simulink model "SingleInverterInfBus"  (R2020b)
settings: Solver=FixedStepAuto  StartTime=0.0  StopTime=20  FixedStep=Ts  RelTol=1e-3
values from neighbouring files (symbols this model uses):
  Cdc = 0.125    [Para.m]    (also in Para_VFM_FFL_Inverter.m = 0.101859163579; Para_VFM_FFL_Inverter_v2.m = 0.101859163579)
  Cf = 0.02    [Para.m]    (also in Para_VFM_FFL_Inverter.m; Para_VFM_FFL_Inverter_v2.m)
  Lc = 0.02    [Para.m]    (also in Para_VFM_FFL_Inverter.m; Para_VFM_FFL_Inverter_v2.m)
  Lf = 0.05    [Para.m]    (also in Para_VFM_FFL_Inverter.m; Para_VFM_FFL_Inverter_v2.m)
  m = 5/100    (= 0.05)    [Para.m]    (also in Para_VFM_FFL_Inverter.m; Para_VFM_FFL_Inverter_v2.m)
  Rline = Xline/5    (= 0.19)    [Para.m]    (also in Para_VFM_FFL_Inverter.m; Para_VFM_FFL_Inverter_v2.m)
  Sbase = 1    [Para.m]    (also in Para_VFM_FFL_Inverter.m; Para_VFM_FFL_Inverter_v2.m)
  Ts = 1/Fs    (= 0.0001)    [Para.m]    (also in Para_VFM_FFL_Inverter.m; Para_VFM_FFL_Inverter_v2.m = 5e-05)
  Vbase = 1    [Para.m]    (also in Para_VFM_FFL_Inverter.m; Para_VFM_FFL_Inverter_v2.m)
  vdc_ref = 2.5    [Para.m]    (also in Para_VFM_FFL_Inverter.m; Para_VFM_FFL_Inverter_v2.m)
  w_droop = 1*2*pi    (= 6.28318530718)    [Para.m]    (also in Para_VFM_FFL_Inverter.m = 31.4159265359; Para_VFM_FFL_Inverter_v2.m = 31.4159265359)
  w_i = 600*2*pi    (= 3769.91118431)    [Para.m]    (also in Para_VFM_FFL_Inverter.m; Para_VFM_FFL_Inverter_v2.m)
  w_pll = 15*2*pi    (= 94.2477796077)    [Para.m]    (also in Para_VFM_FFL_Inverter.m; Para_VFM_FFL_Inverter_v2.m)
  w_tau = 200*2*pi    (= 1256.63706144)    [Para.m]    (also in Para_VFM_FFL_Inverter.m; Para_VFM_FFL_Inverter_v2.m)
  w_v = 300*2*pi    (= 1884.95559215)    [Para.m]    (also in Para_VFM_FFL_Inverter.m; Para_VFM_FFL_Inverter_v2.m)
  w_vdc = 5*2*pi    (= 31.4159265359)    [Para.m]    (also in Para_VFM_FFL_Inverter.m; Para_VFM_FFL_Inverter_v2.m)
  Wbase = 2*pi*50    (= 314.159265359)    [Para.m]    (also in Para_VFM_FFL_Inverter.m; Para_VFM_FFL_Inverter_v2.m)
  Xline = 0.95    [Para.m]    (also in Para_VFM_FFL_Inverter.m; Para_VFM_FFL_Inverter_v2.m)
  Zbase = Vbase/Ibase    (= 1)    [Para.m]    (also in Para_VFM_FFL_Inverter.m; Para_VFM_FFL_Inverter_v2.m)
undefined symbols (not defined in the file or in its folder): DiscIntNeverNeededParam, initial
libraries: powerlib x282, SimplusGT x7
(part 3 of 8)

== system SingleInverterInfBus/Subsystem3 ==
  In1 : Inport
  Constant : Constant  Value=pi/2
  Constant2 : Constant  Value=2*pi
  Math Function1 : Math  Operator=mod  SignedPower=on  SaturateOnIntegerOverflow=on
  Sum1 : Sum  Inputs=|+-
  Sum3 : Sum  Inputs=|++
  Out1 : Outport
  wires:
  Sum3/1 -> Math Function1/1
  Constant2/1 -> Math Function1/2
  In1/1 -> Sum3/1
  Constant/1 -> Sum3/2, Sum1/2
  Math Function1/1 -> Sum1/1
  Sum1/1 -> Out1/1

== system SingleInverterInfBus/Subsystem4 ==
  In1 : Inport
  Constant : Constant  Value=pi/2
  Constant2 : Constant  Value=2*pi
  Math Function1 : Math  Operator=mod  SignedPower=on  SaturateOnIntegerOverflow=on
  Sum1 : Sum  Inputs=|+-
  Sum3 : Sum  Inputs=|++
  Out1 : Outport
  wires:
  Sum3/1 -> Math Function1/1
  Constant2/1 -> Math Function1/2
  In1/1 -> Sum3/1
  Constant/1 -> Sum1/2, Sum3/2
  Math Function1/1 -> Sum1/1
  Sum1/1 -> Out1/1

== system SingleInverterInfBus/Subsystem5 ==
  In1 : Inport
  Transfer Fcn : TransferFcn  Numerator=[1 0 0]  Denominator=[1 kp ki]
  Out1 : Outport
  wires:
  Transfer Fcn/1 -> Out1/1
  In1/1 -> Transfer Fcn/1

== system SingleInverterInfBus/Subsystem6 ==
  In1 : Inport
  Transfer Fcn : TransferFcn  Numerator=[1 kd*ki 0]  Denominator=[1 kd*ki ki]
  Out1 : Outport
  wires:
  Transfer Fcn/1 -> Out1/1
  In1/1 -> Transfer Fcn/1

== system SingleInverterInfBus/Subsystem7 ==
  In1 : Inport
  Transfer Fcn : TransferFcn  Numerator=[1 0]  Denominator=[1 kp ki]
  Out1 : Outport
  wires:
  Transfer Fcn/1 -> Out1/1
  In1/1 -> Transfer Fcn/1

== system SingleInverterInfBus/Subsystem8 ==
  In1 : Inport
  Transfer Fcn : TransferFcn  Numerator=[1 kd*ki]  Denominator=[1 kd*ki ki]
  Out1 : Outport
  wires:
  Transfer Fcn/1 -> Out1/1
  In1/1 -> Transfer Fcn/1

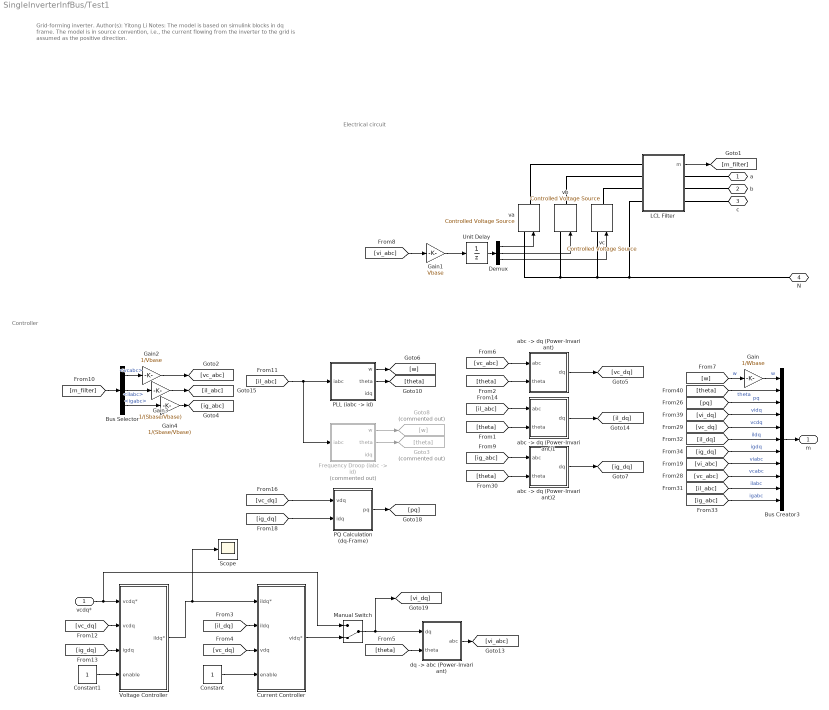
== system SingleInverterInfBus/Test1 ==
  note: Grid-forming inverter.
      |
      | Author(s): Yitong Li
      |
      | Notes:
      |
      | The model is based on simulink blocks in dq frame.
      |
      | The model is in source convention, i.e., the current flowing from the inverter to the grid is assumed as the positive direction.
  note: Electrical circuit
  note: Controller
  vcdq* : Inport
  Bus Creator3 : BusCreator  Inputs=11
  Bus Selector : BusSelector  OutputSignals=vcabc,ilabc,igabc
  Constant : Constant
  Constant1 : Constant
  Current Controller : Subsystem  mask{Ts=Ts, Wbase=Wbase, Lf=Lf/Wbase, Kg=0, Kp=w_i*Lf/Wbase, Ki=w_i*w_i/4*Lf/Wbase, xdmax=inf, xqmax=inf, Kcd=0}
      mask prompts: Ts "Sampling Time (s)"; Wbase "Base Angular Frequency (rad/s)"; Lf "Inductance"; Kg "Estimator Gain"; Kp "Proportional Gain"; Ki "Integral Gain"; xdmax "Voltage D Limit"; xqmax "Voltage Q Limit"; Kcd "Cross Decoupling Gain"
  Demux : Demux  Outputs=3
  "Frequency Droop (iabc -> id)" : Subsystem  Commented=on  AncestorBlock=|  mask{Ts=Ts, Sbase=Sbase, Vbase=Vbase, Wbase=Wbase, m=5/100, w_tau=15*2*pi, theta0=0, i0=0, w0=1}
      | SimplusGT/Frequency Droop
      | (iabc -> id)
      mask prompts: Ts "Ts (s), samping period"; Sbase "Sbase (VA), base power"; Vbase "Vbase (V), base voltage"; Wbase "Wbase (rad/s), base angular frequency"; m "m (pu), droop gain"; w_tau "w_tau (rad/s), low-pass filter bandwidth"; theta0 "theta0 (rad), initial angle"; i0 "i0 (pu), current setting point"; w0 "w0 (pu), frequency setting point"
  Gain : Gain  Gain=1/Wbase
  Gain1 : Gain  Gain=Vbase
  Gain2 : Gain  Gain=1/Vbase
  Gain3 : Gain  Gain=1/(Sbase/Vbase)
  Gain4 : Gain  Gain=1/(Sbase/Vbase)
  Goto3 : Goto  Commented=on  GotoTag=theta
  Goto8 : Goto  Commented=on  GotoTag=w
  LCL Filter : Subsystem  AncestorBlock=SimplexPS/LCL Filter  mask{Lf=Lf*(Vbase^2/Sbase)/Wbase, Rf=Lf*(Vbase^2/Sbase)/5, Lc=Lc*(Vbase^2/Sbase)/Wbase, Rc=Lc*(Vbase^2/Sbase)/5, Cf=Cf*(Sbase/Vbase^2)/Wbase, Rd=1e-5*(Vbase^2/Sbase)}
      mask prompts: Lf "Lf (H)"; Rf "Rf (Ohm)"; Lc "Lc (H)"; Rc "Rc (Ohm)"; Cf "Cf (F)"; Rd "Rd (Ohm)"
  Manual Switch : ManualSwitch  CurrentSetting=0
  "PLL (iabc -> id)" : Subsystem  mask{Ts=Ts, Ibase=Sbase/Vbase, Wbase=Wbase, w_pll=0, w_tau=0, theta0=0}
      mask prompts: Ts "Ts (s), sampling period"; Ibase "Ibase (V), base current"; Wbase "Wbase (rad/s), base angular frequency"; w_pll "w_pll (rad/s), PLL bandwidth"; w_tau "w_tau (rad/s), low-pass filter bandwidth"; theta0 "theta0 (rad), initial angle"
  PQ Calculation (dq-Frame) : Subsystem  AncestorBlock=|
      | SimplusGT/PQ Calculation
      | (dq-Frame)
  Scope : Scope
  Unit Delay : UnitDelay  SampleTime=-1  HasFrameUpgradeWarning=on
  Voltage Controller : Subsystem  mask{Ts=Ts, Wbase=Wbase, Cf=Cf/Wbase, Kg=0, Kp=w_v*Cf/Wbase, Ki=w_v*w_v/4*Cf/Wbase*50, xdmax=inf, xqmax=inf, Kcd=0}
      mask prompts: Ts "Sampling Time (s)"; Wbase "Base Angular Frequency (rad/s)"; Cf "Capacitance"; Kg "Estimator Gain"; Kp "Proportional Gain"; Ki "Integral Gain"; xdmax "Current D Limit"; xqmax "Current Q Limit"; Kcd "Cross Decoupling Gain"
  "abc -> dq (Power-Invariant)" : Subsystem  AncestorBlock=|
      | SimplusGT/abc -> dq
      | (Power-Invariant)
  "abc -> dq (Power-Invariant)1" : Subsystem  AncestorBlock=|
      | SimplusGT/abc -> dq
      | (Power-Invariant)
  "abc -> dq (Power-Invariant)2" : Subsystem  AncestorBlock=|
      | SimplusGT/abc -> dq
      | (Power-Invariant)
  "dq -> abc (Power-Invariant)" : Subsystem  AncestorBlock=|
      | SimplusGT/dq -> abc
      | (Power-Invariant)
  va : powerlib/Electrical Sources/Controlled Voltage Source  Initialize=on  Source_Type=AC  Amplitude=0  Phase=0  Frequency=0  Measurements=None
  vb : powerlib/Electrical Sources/Controlled Voltage Source  Initialize=on  Source_Type=AC  Amplitude=0  Phase=0  Frequency=0  Measurements=None
  vc : powerlib/Electrical Sources/Controlled Voltage Source  Initialize=on  Source_Type=AC  Amplitude=0  Phase=0  Frequency=0  Measurements=None
  a : PMIOPort  Side=Right
  b : PMIOPort  Port=2  Side=Right
  c : PMIOPort  Port=3  Side=Right
  N : PMIOPort  Port=4  Side=Right
  m : Outport
  wires:
  Gain1/1 -> Unit Delay/1
  [vi_abc] -> Gain1/1
  Gain4/1 -> [ig_abc]
  Gain3/1 -> [il_abc]
  Gain2/1 -> [vc_abc]
  [ig_dq] -> Voltage Controller/3(igdq)
  [vc_dq] -> Voltage Controller/2(vcdq)
  Constant1/1 -> Voltage Controller/4(enable)
  Voltage Controller/1(ildq*) -> Scope/1, Current Controller/1(iIdq*)
  vcdq*/1 -> Manual Switch/1, Voltage Controller/1(vcdq*)
  [ig_abc] -> Bus Creator3/11  "igabc"
  [il_abc] -> Bus Creator3/10  "ilabc"
  [vc_abc] -> Bus Creator3/9  "vcabc"
  [vi_abc] -> Bus Creator3/8  "viabc"
  [ig_dq] -> Bus Creator3/7  "igdq"
  [il_dq] -> Bus Creator3/6  "ildq"
  [vc_dq] -> Bus Creator3/5  "vcdq"
  [vi_dq] -> Bus Creator3/4  "vidq"
  [pq] -> Bus Creator3/3  "pq"
  [theta] -> Bus Creator3/2  "theta"
  Gain/1 -> Bus Creator3/1  "w"
  [w] -> Gain/1  "w"
  Bus Selector/1 -> Gain2/1  "<vcabc>"
  Unit Delay/1 -> Demux/1
  [m_filter] -> Bus Selector/1
  "abc -> dq (Power-Invariant)1"/1(dq) -> [il_dq]
  "abc -> dq (Power-Invariant)2"/1(dq) -> [ig_dq]
  "abc -> dq (Power-Invariant)"/1(dq) -> [vc_dq]
  [il_dq] -> Current Controller/2(iIdq)
  [ig_dq] -> PQ Calculation (dq-Frame)/2(idq)
  PQ Calculation (dq-Frame)/1(pq) -> [pq]
  [vc_dq] -> PQ Calculation (dq-Frame)/1(vdq)
  [theta] -> "dq -> abc (Power-Invariant)"/2(theta)
  [vc_dq] -> Current Controller/3(vdq)
  Constant/1 -> Current Controller/4(enable)
  Bus Selector/2 -> Gain3/1  "<ilabc>"
  Bus Selector/3 -> Gain4/1  "<igabc>"
  [theta] -> "abc -> dq (Power-Invariant)2"/2(theta)
  [ig_abc] -> "abc -> dq (Power-Invariant)2"/1(abc)
  [il_abc] -> "abc -> dq (Power-Invariant)1"/1(abc)
  [vc_abc] -> "abc -> dq (Power-Invariant)"/1(abc)
  [theta] -> "abc -> dq (Power-Invariant)1"/2(theta)
  [theta] -> "abc -> dq (Power-Invariant)"/2(theta)
  Demux/3 -> vc/1
  Demux/2 -> vb/1
  Demux/1 -> va/1
  LCL Filter/1(m) -> [m_filter]
  Bus Creator3/1 -> m/1
  "dq -> abc (Power-Invariant)"/1(abc) -> [vi_abc]
  Current Controller/1(vidq*) -> Manual Switch/2
  Manual Switch/1 -> [vi_dq], "dq -> abc (Power-Invariant)"/1(dq)
  "PLL (iabc -> id)"/1(w) -> [w]
  "PLL (iabc -> id)"/2(theta) -> [theta]
  [il_abc] -> "Frequency Droop (iabc -> id)"/1(iabc), "PLL (iabc -> id)"/1(iabc)
  "Frequency Droop (iabc -> id)"/1(w) -> Goto8/1
  "Frequency Droop (iabc -> id)"/2(theta) -> Goto3/1
  connections:
  LCL Filter/LConn3 -- vc/RConn1
  va/LConn1 -- vb/LConn1 -- vc/LConn1 -- LCL Filter/LConn4 -- N/RConn1
  LCL Filter/RConn3 -- c/RConn1
  LCL Filter/RConn2 -- b/RConn1
  LCL Filter/RConn1 -- a/RConn1
  LCL Filter/LConn1 -- va/RConn1
  LCL Filter/LConn2 -- vb/RConn1

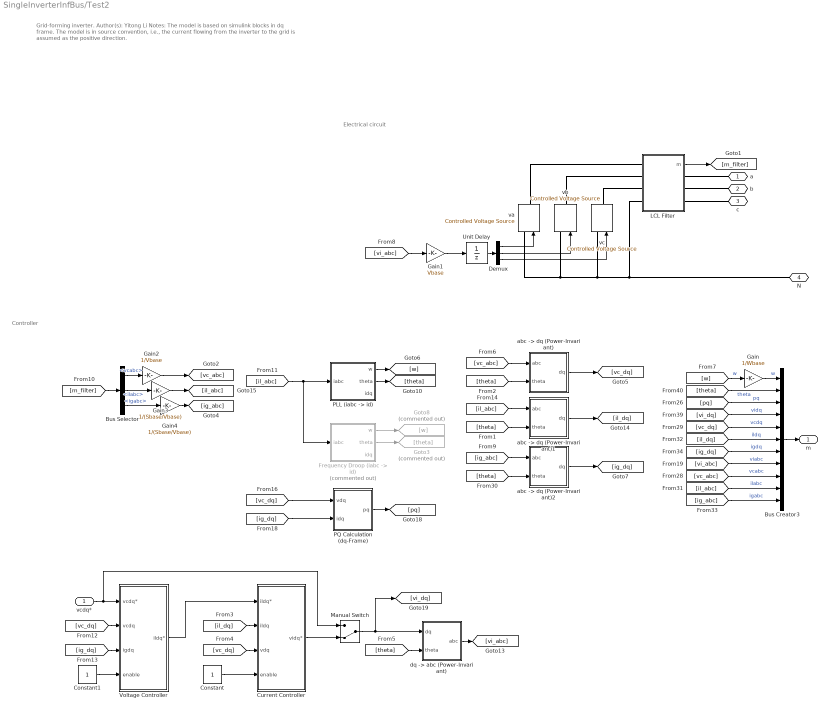
== system SingleInverterInfBus/Test2 ==
  note: Grid-forming inverter.
      |
      | Author(s): Yitong Li
      |
      | Notes:
      |
      | The model is based on simulink blocks in dq frame.
      |
      | The model is in source convention, i.e., the current flowing from the inverter to the grid is assumed as the positive direction.
  note: Electrical circuit
  note: Controller
  vcdq* : Inport
  Bus Creator3 : BusCreator  Inputs=11
  Bus Selector : BusSelector  OutputSignals=vcabc,ilabc,igabc
  Constant : Constant
  Constant1 : Constant
  Current Controller : Subsystem  mask{Ts=Ts, Wbase=Wbase, Lf=Lf/Wbase, Kg=0, Kp=w_i*Lf/Wbase, Ki=w_i*w_i/4*Lf/Wbase, xdmax=inf, xqmax=inf, Kcd=0}
      mask prompts: Ts "Sampling Time (s)"; Wbase "Base Angular Frequency (rad/s)"; Lf "Inductance"; Kg "Estimator Gain"; Kp "Proportional Gain"; Ki "Integral Gain"; xdmax "Voltage D Limit"; xqmax "Voltage Q Limit"; Kcd "Cross Decoupling Gain"
  Demux : Demux  Outputs=3
  "Frequency Droop (iabc -> id)" : Subsystem  Commented=on  AncestorBlock=|  mask{Ts=Ts, Sbase=Sbase, Vbase=Vbase, Wbase=Wbase, m=5/100, w_tau=15*2*pi, theta0=0, i0=0, w0=1}
      | SimplusGT/Frequency Droop
      | (iabc -> id)
      mask prompts: Ts "Ts (s), samping period"; Sbase "Sbase (VA), base power"; Vbase "Vbase (V), base voltage"; Wbase "Wbase (rad/s), base angular frequency"; m "m (pu), droop gain"; w_tau "w_tau (rad/s), low-pass filter bandwidth"; theta0 "theta0 (rad), initial angle"; i0 "i0 (pu), current setting point"; w0 "w0 (pu), frequency setting point"
  Gain : Gain  Gain=1/Wbase
  Gain1 : Gain  Gain=Vbase
  Gain2 : Gain  Gain=1/Vbase
  Gain3 : Gain  Gain=1/(Sbase/Vbase)
  Gain4 : Gain  Gain=1/(Sbase/Vbase)
  Goto3 : Goto  Commented=on  GotoTag=theta
  Goto8 : Goto  Commented=on  GotoTag=w
  LCL Filter : Subsystem  AncestorBlock=SimplexPS/LCL Filter  mask{Lf=Lf*(Vbase^2/Sbase)/Wbase, Rf=Lf*(Vbase^2/Sbase)/5, Lc=Lc*(Vbase^2/Sbase)/Wbase, Rc=Lc*(Vbase^2/Sbase)/5, Cf=Cf*(Sbase/Vbase^2)/Wbase, Rd=1e-5*(Vbase^2/Sbase)}
      mask prompts: Lf "Lf (H)"; Rf "Rf (Ohm)"; Lc "Lc (H)"; Rc "Rc (Ohm)"; Cf "Cf (F)"; Rd "Rd (Ohm)"
  Manual Switch : ManualSwitch  CurrentSetting=0
  "PLL (iabc -> id)" : Subsystem  mask{Ts=Ts, Ibase=Sbase/Vbase, Wbase=Wbase, w_pll=5*2*pi, w_tau=15*2*pi, theta0=0}
      mask prompts: Ts "Ts (s), sampling period"; Ibase "Ibase (V), base current"; Wbase "Wbase (rad/s), base angular frequency"; w_pll "w_pll (rad/s), PLL bandwidth"; w_tau "w_tau (rad/s), low-pass filter bandwidth"; theta0 "theta0 (rad), initial angle"
  PQ Calculation (dq-Frame) : Subsystem  AncestorBlock=|
      | SimplusGT/PQ Calculation
      | (dq-Frame)
  Unit Delay : UnitDelay  SampleTime=-1  HasFrameUpgradeWarning=on
  Voltage Controller : Subsystem  mask{Ts=Ts, Wbase=Wbase, Cf=Cf/Wbase, Kg=0, Kp=w_v*Cf/Wbase, Ki=w_v*w_v/4*Cf/Wbase*20, xdmax=inf, xqmax=inf, Kcd=0}
      mask prompts: Ts "Sampling Time (s)"; Wbase "Base Angular Frequency (rad/s)"; Cf "Capacitance"; Kg "Estimator Gain"; Kp "Proportional Gain"; Ki "Integral Gain"; xdmax "Current D Limit"; xqmax "Current Q Limit"; Kcd "Cross Decoupling Gain"
  "abc -> dq (Power-Invariant)" : Subsystem  AncestorBlock=|
      | SimplusGT/abc -> dq
      | (Power-Invariant)
  "abc -> dq (Power-Invariant)1" : Subsystem  AncestorBlock=|
      | SimplusGT/abc -> dq
      | (Power-Invariant)
  "abc -> dq (Power-Invariant)2" : Subsystem  AncestorBlock=|
      | SimplusGT/abc -> dq
      | (Power-Invariant)
  "dq -> abc (Power-Invariant)" : Subsystem  AncestorBlock=|
      | SimplusGT/dq -> abc
      | (Power-Invariant)
  va : powerlib/Electrical Sources/Controlled Voltage Source  Initialize=on  Source_Type=AC  Amplitude=0  Phase=0  Frequency=0  Measurements=None
  vb : powerlib/Electrical Sources/Controlled Voltage Source  Initialize=on  Source_Type=AC  Amplitude=0  Phase=0  Frequency=0  Measurements=None
  vc : powerlib/Electrical Sources/Controlled Voltage Source  Initialize=on  Source_Type=AC  Amplitude=0  Phase=0  Frequency=0  Measurements=None
  a : PMIOPort  Side=Right
  b : PMIOPort  Port=2  Side=Right
  c : PMIOPort  Port=3  Side=Right
  N : PMIOPort  Port=4  Side=Right
  m : Outport
  wires:
  Gain1/1 -> Unit Delay/1
  [vi_abc] -> Gain1/1
  Gain4/1 -> [ig_abc]
  Gain3/1 -> [il_abc]
  Gain2/1 -> [vc_abc]
  [ig_dq] -> Voltage Controller/3(igdq)
  [vc_dq] -> Voltage Controller/2(vcdq)
  Constant1/1 -> Voltage Controller/4(enable)
  Voltage Controller/1(ildq*) -> Current Controller/1(iIdq*)
  vcdq*/1 -> Manual Switch/1, Voltage Controller/1(vcdq*)
  [ig_abc] -> Bus Creator3/11  "igabc"
  [il_abc] -> Bus Creator3/10  "ilabc"
  [vc_abc] -> Bus Creator3/9  "vcabc"
  [vi_abc] -> Bus Creator3/8  "viabc"
  [ig_dq] -> Bus Creator3/7  "igdq"
  [il_dq] -> Bus Creator3/6  "ildq"
  [vc_dq] -> Bus Creator3/5  "vcdq"
  [vi_dq] -> Bus Creator3/4  "vidq"
  [pq] -> Bus Creator3/3  "pq"
  [theta] -> Bus Creator3/2  "theta"
  Gain/1 -> Bus Creator3/1  "w"
  [w] -> Gain/1  "w"
  Bus Selector/1 -> Gain2/1  "<vcabc>"
  Unit Delay/1 -> Demux/1
  [m_filter] -> Bus Selector/1
  "abc -> dq (Power-Invariant)1"/1(dq) -> [il_dq]
  "abc -> dq (Power-Invariant)2"/1(dq) -> [ig_dq]
  "abc -> dq (Power-Invariant)"/1(dq) -> [vc_dq]
  [il_dq] -> Current Controller/2(iIdq)
  [ig_dq] -> PQ Calculation (dq-Frame)/2(idq)
  PQ Calculation (dq-Frame)/1(pq) -> [pq]
  [vc_dq] -> PQ Calculation (dq-Frame)/1(vdq)
  [theta] -> "dq -> abc (Power-Invariant)"/2(theta)
  [vc_dq] -> Current Controller/3(vdq)
  Constant/1 -> Current Controller/4(enable)
  Bus Selector/2 -> Gain3/1  "<ilabc>"
  Bus Selector/3 -> Gain4/1  "<igabc>"
  [theta] -> "abc -> dq (Power-Invariant)2"/2(theta)
  [ig_abc] -> "abc -> dq (Power-Invariant)2"/1(abc)
  [il_abc] -> "abc -> dq (Power-Invariant)1"/1(abc)
  [vc_abc] -> "abc -> dq (Power-Invariant)"/1(abc)
  [theta] -> "abc -> dq (Power-Invariant)1"/2(theta)
  [theta] -> "abc -> dq (Power-Invariant)"/2(theta)
  Demux/3 -> vc/1
  Demux/2 -> vb/1
  Demux/1 -> va/1
  LCL Filter/1(m) -> [m_filter]
  Bus Creator3/1 -> m/1
  "dq -> abc (Power-Invariant)"/1(abc) -> [vi_abc]
  Current Controller/1(vidq*) -> Manual Switch/2
  Manual Switch/1 -> [vi_dq], "dq -> abc (Power-Invariant)"/1(dq)
  "PLL (iabc -> id)"/1(w) -> [w]
  "PLL (iabc -> id)"/2(theta) -> [theta]
  [il_abc] -> "Frequency Droop (iabc -> id)"/1(iabc), "PLL (iabc -> id)"/1(iabc)
  "Frequency Droop (iabc -> id)"/1(w) -> Goto8/1
  "Frequency Droop (iabc -> id)"/2(theta) -> Goto3/1
  connections:
  LCL Filter/LConn3 -- vc/RConn1
  va/LConn1 -- vb/LConn1 -- vc/LConn1 -- LCL Filter/LConn4 -- N/RConn1
  LCL Filter/RConn3 -- c/RConn1
  LCL Filter/RConn2 -- b/RConn1
  LCL Filter/RConn1 -- a/RConn1
  LCL Filter/LConn1 -- va/RConn1
  LCL Filter/LConn2 -- vb/RConn1

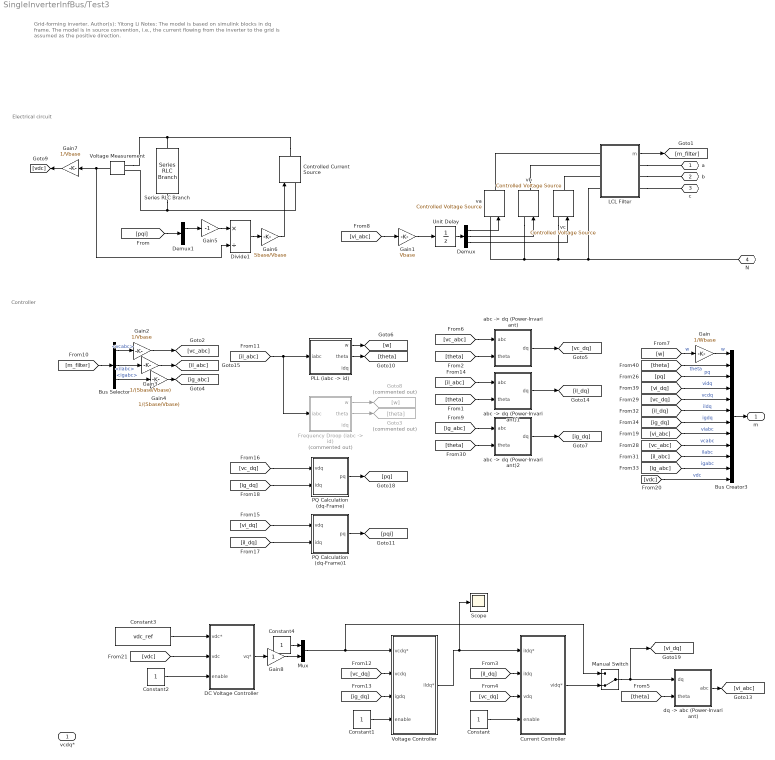
== system SingleInverterInfBus/Test3 ==
  note: Grid-forming inverter.
      |
      | Author(s): Yitong Li
      |
      | Notes:
      |
      | The model is based on simulink blocks in dq frame.
      |
      | The model is in source convention, i.e., the current flowing from the inverter to the grid is assumed as the positive direction.
  note: Electrical circuit
  note: Controller
  vcdq* : Inport
  Bus Creator3 : BusCreator  Inputs=12
  Bus Selector : BusSelector  OutputSignals=vcabc,ilabc,igabc
  Constant{,1..2,4} (4 alike) : Constant
  Constant3 : Constant  Value=vdc_ref
  Controlled Current Source : powerlib/Electrical Sources/Controlled Current Source  Initialize=on  Source_Type=AC  Amplitude=0  Phase=0  Frequency=0  Measurements=None
  Current Controller : Subsystem  mask{Ts=Ts, Wbase=Wbase, Lf=Lf/Wbase, Kg=0, Kp=w_i*Lf/Wbase, Ki=w_i*w_i/4*Lf/Wbase, xdmax=inf, xqmax=inf, Kcd=0}
      mask prompts: Ts "Sampling Time (s)"; Wbase "Base Angular Frequency (rad/s)"; Lf "Inductance"; Kg "Estimator Gain"; Kp "Proportional Gain"; Ki "Integral Gain"; xdmax "Voltage D Limit"; xqmax "Voltage Q Limit"; Kcd "Cross Decoupling Gain"
  DC Voltage Controller : Subsystem  mask{Ts=Ts, Wbase=Wbase, Kg=0, Kp=vdc_ref*Cdc*w_vdc, Ki=vdc_ref*Cdc*w_vdc^2/4}
      mask prompts: Ts "Sampling Time (s)"; Wbase "Base Angular Frequency (rad/s)"; Kg "Estimator Gain"; Kp "Proportional Gain"; Ki "Integral Gain"
  Demux : Demux  Outputs=3
  Demux1 : Demux  Outputs=2
  Divide1 : Product  Inputs=*/
  "Frequency Droop (iabc -> id)" : Subsystem  Commented=on  AncestorBlock=|  mask{Ts=Ts, Sbase=Sbase, Vbase=Vbase, Wbase=Wbase, m=5/100, w_tau=15*2*pi, theta0=0, i0=0, w0=1}
      | SimplusGT/Frequency Droop
      | (iabc -> id)
      mask prompts: Ts "Ts (s), samping period"; Sbase "Sbase (VA), base power"; Vbase "Vbase (V), base voltage"; Wbase "Wbase (rad/s), base angular frequency"; m "m (pu), droop gain"; w_tau "w_tau (rad/s), low-pass filter bandwidth"; theta0 "theta0 (rad), initial angle"; i0 "i0 (pu), current setting point"; w0 "w0 (pu), frequency setting point"
  Gain : Gain  Gain=1/Wbase
  Gain1 : Gain  Gain=Vbase
  Gain2 : Gain  Gain=1/Vbase
  Gain3 : Gain  Gain=1/(Sbase/Vbase)
  Gain4 : Gain  Gain=1/(Sbase/Vbase)
  Gain5 : Gain  Gain=-1
  Gain6 : Gain  Gain=Sbase/Vbase
  Gain7 : Gain  Gain=1/Vbase
  Gain8 : Gain
  Goto3 : Goto  Commented=on  GotoTag=theta
  Goto8 : Goto  Commented=on  GotoTag=w
  LCL Filter : Subsystem  AncestorBlock=SimplexPS/LCL Filter  mask{Lf=Lf*(Vbase^2/Sbase)/Wbase, Rf=Lf*(Vbase^2/Sbase)/5, Lc=Lc*(Vbase^2/Sbase)/Wbase, Rc=Lc*(Vbase^2/Sbase)/5, Cf=Cf*(Sbase/Vbase^2)/Wbase, Rd=1e-5*(Vbase^2/Sbase)}
      mask prompts: Lf "Lf (H)"; Rf "Rf (Ohm)"; Lc "Lc (H)"; Rc "Rc (Ohm)"; Cf "Cf (F)"; Rd "Rd (Ohm)"
  Manual Switch : ManualSwitch  CurrentSetting=0
  Mux : Mux  Inputs=2
  "PLL (iabc -> id)" : Subsystem  mask{Ts=Ts, Ibase=Sbase/Vbase, Wbase=Wbase, w_pll=0, w_tau=0, theta0=0}
      mask prompts: Ts "Ts (s), sampling period"; Ibase "Ibase (V), base current"; Wbase "Wbase (rad/s), base angular frequency"; w_pll "w_pll (rad/s), PLL bandwidth"; w_tau "w_tau (rad/s), low-pass filter bandwidth"; theta0 "theta0 (rad), initial angle"
  PQ Calculation (dq-Frame) : Subsystem  AncestorBlock=|
      | SimplusGT/PQ Calculation
      | (dq-Frame)
  PQ Calculation (dq-Frame)1 : Subsystem  AncestorBlock=|
      | SimplusGT/PQ Calculation
      | (dq-Frame)
  Scope : Scope
  Series RLC Branch : powerlib/Elements/Series RLC Branch  LConnTagsString=__new0  RConnTagsString=__new0  BranchType=RC  Resistance=1e-9*(Vbase^2/Sbase)  Inductance=1e-3  SetiL0=off  InitialCurrent=0  Capacitance=Cdc*(Sbase/Vbase^2)  Setx0=on  InitialVoltage=Vbase*vdc_ref  Measurements=None
  Unit Delay : UnitDelay  SampleTime=-1  HasFrameUpgradeWarning=on
  Voltage Controller : Subsystem  mask{Ts=Ts, Wbase=Wbase, Cf=Cf/Wbase, Kg=0, Kp=w_v*Cf/Wbase, Ki=w_v*w_v/4*Cf/Wbase*50, xdmax=inf, xqmax=inf, Kcd=0}
      mask prompts: Ts "Sampling Time (s)"; Wbase "Base Angular Frequency (rad/s)"; Cf "Capacitance"; Kg "Estimator Gain"; Kp "Proportional Gain"; Ki "Integral Gain"; xdmax "Current D Limit"; xqmax "Current Q Limit"; Kcd "Cross Decoupling Gain"
  Voltage Measurement : powerlib/Measurements/Voltage Measurement  PhasorSimulation=off  OutputType=Complex  PSBequivalent=0
  "abc -> dq (Power-Invariant)" : Subsystem  AncestorBlock=|
      | SimplusGT/abc -> dq
      | (Power-Invariant)
  "abc -> dq (Power-Invariant)1" : Subsystem  AncestorBlock=|
      | SimplusGT/abc -> dq
      | (Power-Invariant)
  "abc -> dq (Power-Invariant)2" : Subsystem  AncestorBlock=|
      | SimplusGT/abc -> dq
      | (Power-Invariant)
  "dq -> abc (Power-Invariant)" : Subsystem  AncestorBlock=|
      | SimplusGT/dq -> abc
      | (Power-Invariant)
  va : powerlib/Electrical Sources/Controlled Voltage Source  Initialize=on  Source_Type=AC  Amplitude=0  Phase=0  Frequency=0  Measurements=None
  vb : powerlib/Electrical Sources/Controlled Voltage Source  Initialize=on  Source_Type=AC  Amplitude=0  Phase=0  Frequency=0  Measurements=None
  vc : powerlib/Electrical Sources/Controlled Voltage Source  Initialize=on  Source_Type=AC  Amplitude=0  Phase=0  Frequency=0  Measurements=None
  a : PMIOPort  Side=Right
  b : PMIOPort  Port=2  Side=Right
  c : PMIOPort  Port=3  Side=Right
  N : PMIOPort  Port=4  Side=Right
  m : Outport
  wires:
  Gain1/1 -> Unit Delay/1
  [vi_abc] -> Gain1/1
  Gain4/1 -> [ig_abc]
  Gain3/1 -> [il_abc]
  Gain2/1 -> [vc_abc]
  [ig_dq] -> Voltage Controller/3(igdq)
  [vc_dq] -> Voltage Controller/2(vcdq)
  Constant1/1 -> Voltage Controller/4(enable)
  Voltage Controller/1(ildq*) -> Scope/1, Current Controller/1(iIdq*)
  [ig_abc] -> Bus Creator3/11  "igabc"
  [il_abc] -> Bus Creator3/10  "ilabc"
  [vc_abc] -> Bus Creator3/9  "vcabc"
  [vi_abc] -> Bus Creator3/8  "viabc"
  [ig_dq] -> Bus Creator3/7  "igdq"
  [il_dq] -> Bus Creator3/6  "ildq"
  [vc_dq] -> Bus Creator3/5  "vcdq"
  [vi_dq] -> Bus Creator3/4  "vidq"
  [pq] -> Bus Creator3/3  "pq"
  [theta] -> Bus Creator3/2  "theta"
  Gain/1 -> Bus Creator3/1  "w"
  [w] -> Gain/1  "w"
  Bus Selector/1 -> Gain2/1  "<vcabc>"
  Unit Delay/1 -> Demux/1
  [m_filter] -> Bus Selector/1
  "abc -> dq (Power-Invariant)1"/1(dq) -> [il_dq]
  "abc -> dq (Power-Invariant)2"/1(dq) -> [ig_dq]
  "abc -> dq (Power-Invariant)"/1(dq) -> [vc_dq]
  [il_dq] -> Current Controller/2(iIdq)
  [ig_dq] -> PQ Calculation (dq-Frame)/2(idq)
  PQ Calculation (dq-Frame)/1(pq) -> [pq]
  [vc_dq] -> PQ Calculation (dq-Frame)/1(vdq)
  [theta] -> "dq -> abc (Power-Invariant)"/2(theta)
  [vc_dq] -> Current Controller/3(vdq)
  Constant/1 -> Current Controller/4(enable)
  Bus Selector/2 -> Gain3/1  "<ilabc>"
  Bus Selector/3 -> Gain4/1  "<igabc>"
  [theta] -> "abc -> dq (Power-Invariant)2"/2(theta)
  [ig_abc] -> "abc -> dq (Power-Invariant)2"/1(abc)
  [il_abc] -> "abc -> dq (Power-Invariant)1"/1(abc)
  [vc_abc] -> "abc -> dq (Power-Invariant)"/1(abc)
  [theta] -> "abc -> dq (Power-Invariant)1"/2(theta)
  [theta] -> "abc -> dq (Power-Invariant)"/2(theta)
  Demux/3 -> vc/1
  Demux/2 -> vb/1
  Demux/1 -> va/1
  LCL Filter/1(m) -> [m_filter]
  Bus Creator3/1 -> m/1
  "dq -> abc (Power-Invariant)"/1(abc) -> [vi_abc]
  Current Controller/1(vidq*) -> Manual Switch/2
  Manual Switch/1 -> [vi_dq], "dq -> abc (Power-Invariant)"/1(dq)
  "PLL (iabc -> id)"/1(w) -> [w]
  "PLL (iabc -> id)"/2(theta) -> [theta]
  [il_abc] -> "Frequency Droop (iabc -> id)"/1(iabc), "PLL (iabc -> id)"/1(iabc)
  "Frequency Droop (iabc -> id)"/1(w) -> Goto8/1
  "Frequency Droop (iabc -> id)"/2(theta) -> Goto3/1
  Divide1/1 -> Gain6/1
  Gain6/1 -> Controlled Current Source/1
  Gain7/1 -> [vdc]
  Demux1/1 -> Gain5/1
  Gain5/1 -> Divide1/1
  [pqi] -> Demux1/1
  Voltage Measurement/1 -> Gain7/1, Divide1/2
  PQ Calculation (dq-Frame)1/1(pq) -> [pqi]
  [il_dq] -> PQ Calculation (dq-Frame)1/2(idq)
  [vi_dq] -> PQ Calculation (dq-Frame)1/1(vdq)
  Constant4/1 -> Mux/1
  DC Voltage Controller/1(vq*) -> Gain8/1
  Gain8/1 -> Mux/2
  Constant2/1 -> DC Voltage Controller/3(enable)
  Constant3/1 -> DC Voltage Controller/1(vdc*)
  [vdc] -> DC Voltage Controller/2(vdc)
  Mux/1 -> Manual Switch/1, Voltage Controller/1(vcdq*)
  [vdc] -> Bus Creator3/12  "vdc"
  connections:
  LCL Filter/LConn3 -- vc/RConn1
  va/LConn1 -- vb/LConn1 -- vc/LConn1 -- LCL Filter/LConn4 -- N/RConn1
  LCL Filter/RConn3 -- c/RConn1
  LCL Filter/RConn2 -- b/RConn1
  LCL Filter/RConn1 -- a/RConn1
  LCL Filter/LConn1 -- va/RConn1
  LCL Filter/LConn2 -- vb/RConn1
  Controlled Current Source/LConn1 -- Series RLC Branch/RConn1 -- Voltage Measurement/LConn2
  Controlled Current Source/RConn1 -- Series RLC Branch/LConn1 -- Voltage Measurement/LConn1

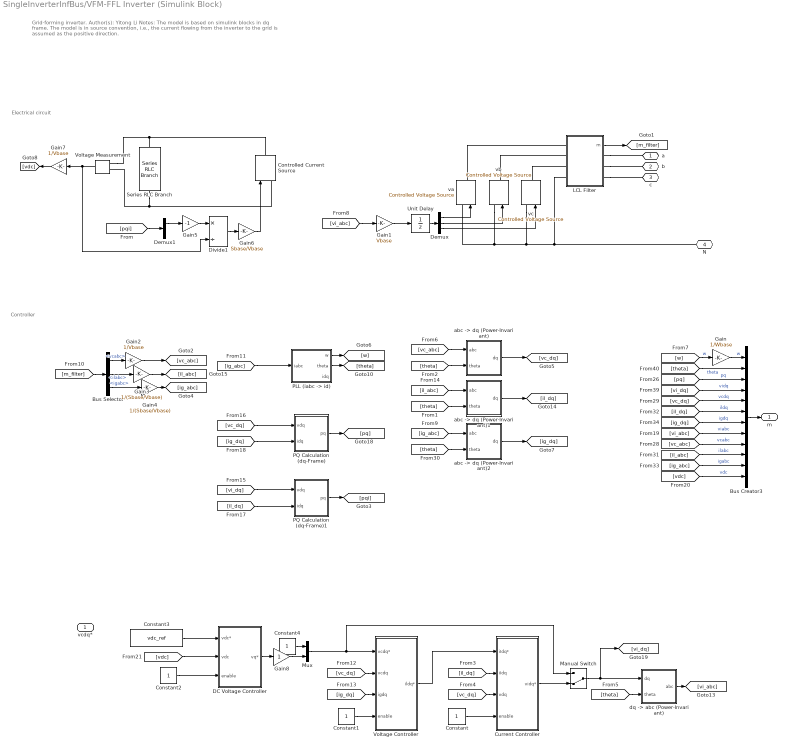
== system SingleInverterInfBus/VFM-FFL Inverter (Simulink Block) ==
  note: Grid-forming inverter.
      |
      | Author(s): Yitong Li
      |
      | Notes:
      |
      | The model is based on simulink blocks in dq frame.
      |
      | The model is in source convention, i.e., the current flowing from the inverter to the grid is assumed as the positive direction.
  note: Electrical circuit
  note: Controller
  vcdq* : Inport
  Bus Creator3 : BusCreator  Inputs=12
  Bus Selector : BusSelector  OutputSignals=vcabc,ilabc,igabc
  Constant{,1..2,4} (4 alike) : Constant
  Constant3 : Constant  Value=vdc_ref
  Controlled Current Source : powerlib/Electrical Sources/Controlled Current Source  Initialize=on  Source_Type=AC  Amplitude=0  Phase=0  Frequency=0  Measurements=None
  Current Controller : Subsystem  mask{Ts=Ts, Wbase=Wbase, Lf=Lf/Wbase, Kg=0, Kp=w_i*Lf/Wbase, Ki=w_i*w_i/4*Lf/Wbase, xdmax=inf, xqmax=inf, Kcd=0}
      mask prompts: Ts "Sampling Time (s)"; Wbase "Base Angular Frequency (rad/s)"; Lf "Inductance"; Kg "Estimator Gain"; Kp "Proportional Gain"; Ki "Integral Gain"; xdmax "Voltage D Limit"; xqmax "Voltage Q Limit"; Kcd "Cross Decoupling Gain"
  DC Voltage Controller : Subsystem  mask{Ts=Ts, Wbase=Wbase, Kg=0, Kp=vdc_ref*Cdc*w_vdc, Ki=vdc_ref*Cdc*w_vdc^2/4}
      mask prompts: Ts "Sampling Time (s)"; Wbase "Base Angular Frequency (rad/s)"; Kg "Estimator Gain"; Kp "Proportional Gain"; Ki "Integral Gain"
  Demux : Demux  Outputs=3
  Demux1 : Demux  Outputs=2
  Divide1 : Product  Inputs=*/
  Gain : Gain  Gain=1/Wbase
  Gain1 : Gain  Gain=Vbase
  Gain2 : Gain  Gain=1/Vbase
  Gain3 : Gain  Gain=1/(Sbase/Vbase)
  Gain4 : Gain  Gain=1/(Sbase/Vbase)
  Gain5 : Gain  Gain=-1
  Gain6 : Gain  Gain=Sbase/Vbase
  Gain7 : Gain  Gain=1/Vbase
  Gain8 : Gain
  LCL Filter : Subsystem  AncestorBlock=SimplexPS/LCL Filter  mask{Lf=wLf*(Vbase^2/Sbase)/Wbase, Rf=wLf*(Vbase^2/Sbase)/5, Lc=wLc*(Vbase^2/Sbase)/Wbase, Rc=wLc*(Vbase^2/Sbase)/5, Cf=wCf*(Sbase/Vbase^2)/Wbase, Rd=1e-9*(Vbase^2/Sbase)}
      mask prompts: Lf "Lf (H)"; Rf "Rf (Ohm)"; Lc "Lc (H)"; Rc "Rc (Ohm)"; Cf "Cf (F)"; Rd "Rd (Ohm)"
  Manual Switch : ManualSwitch  CurrentSetting=0
  Mux : Mux  Inputs=2
  "PLL (iabc -> id)" : Subsystem  mask{Ts=Ts, Ibase=Sbase/Vbase, Wbase=Wbase, w_pll=w_pll, w_tau=w_tau, theta0=0}
      mask prompts: Ts "Ts (s), sampling period"; Ibase "Ibase (V), base current"; Wbase "Wbase (rad/s), base angular frequency"; w_pll "w_pll (rad/s), PLL bandwidth"; w_tau "w_tau (rad/s), low-pass filter bandwidth"; theta0 "theta0 (rad), initial angle"
  PQ Calculation (dq-Frame) : Subsystem  AncestorBlock=|
      | SimplusGT/PQ Calculation
      | (dq-Frame)
  PQ Calculation (dq-Frame)1 : Subsystem  AncestorBlock=|
      | SimplusGT/PQ Calculation
      | (dq-Frame)
  Series RLC Branch : powerlib/Elements/Series RLC Branch  LConnTagsString=__new0  RConnTagsString=__new0  BranchType=RC  Resistance=1e-9*(Vbase^2/Sbase)  Inductance=1e-3  SetiL0=off  InitialCurrent=0  Capacitance=Cdc*(Sbase/Vbase^2)  Setx0=on  InitialVoltage=Vbase*vdc_ref  Measurements=None
  Unit Delay : UnitDelay  SampleTime=-1  HasFrameUpgradeWarning=on
  Voltage Controller : Subsystem  mask{Ts=Ts, Wbase=Wbase, Cf=Cf/Wbase, Kg=0, Kp=w_v*Cf/Wbase, Ki=w_v*w_v/4*Cf/Wbase*20, xdmax=inf, xqmax=inf, Kcd=0}
      mask prompts: Ts "Sampling Time (s)"; Wbase "Base Angular Frequency (rad/s)"; Cf "Capacitance"; Kg "Estimator Gain"; Kp "Proportional Gain"; Ki "Integral Gain"; xdmax "Current D Limit"; xqmax "Current Q Limit"; Kcd "Cross Decoupling Gain"
  Voltage Measurement : powerlib/Measurements/Voltage Measurement  PhasorSimulation=off  OutputType=Complex  PSBequivalent=0
  "abc -> dq (Power-Invariant)" : Subsystem  AncestorBlock=|
      | SimplusGT/abc -> dq
      | (Power-Invariant)
  "abc -> dq (Power-Invariant)1" : Subsystem  AncestorBlock=|
      | SimplusGT/abc -> dq
      | (Power-Invariant)
  "abc -> dq (Power-Invariant)2" : Subsystem  AncestorBlock=|
      | SimplusGT/abc -> dq
      | (Power-Invariant)
  "dq -> abc (Power-Invariant)" : Subsystem  AncestorBlock=|
      | SimplusGT/dq -> abc
      | (Power-Invariant)
  va : powerlib/Electrical Sources/Controlled Voltage Source  Initialize=on  Source_Type=AC  Amplitude=0  Phase=0  Frequency=0  Measurements=None
  vb : powerlib/Electrical Sources/Controlled Voltage Source  Initialize=on  Source_Type=AC  Amplitude=0  Phase=0  Frequency=0  Measurements=None
  vc : powerlib/Electrical Sources/Controlled Voltage Source  Initialize=on  Source_Type=AC  Amplitude=0  Phase=0  Frequency=0  Measurements=None
  a : PMIOPort  Side=Right
  b : PMIOPort  Port=2  Side=Right
  c : PMIOPort  Port=3  Side=Right
  N : PMIOPort  Port=4  Side=Right
  m : Outport
  wires:
  Gain1/1 -> Unit Delay/1
  [vi_abc] -> Gain1/1
  Gain4/1 -> [ig_abc]
  Gain3/1 -> [il_abc]
  Gain2/1 -> [vc_abc]
  [ig_dq] -> Voltage Controller/3(igdq)
  [vc_dq] -> Voltage Controller/2(vcdq)
  Constant1/1 -> Voltage Controller/4(enable)
  Voltage Controller/1(ildq*) -> Current Controller/1(iIdq*)
  [ig_abc] -> Bus Creator3/11  "igabc"
  [il_abc] -> Bus Creator3/10  "ilabc"
  [vc_abc] -> Bus Creator3/9  "vcabc"
  [vi_abc] -> Bus Creator3/8  "viabc"
  [ig_dq] -> Bus Creator3/7  "igdq"
  [il_dq] -> Bus Creator3/6  "ildq"
  [vc_dq] -> Bus Creator3/5  "vcdq"
  [vi_dq] -> Bus Creator3/4  "vidq"
  [pq] -> Bus Creator3/3  "pq"
  [theta] -> Bus Creator3/2  "theta"
  Gain/1 -> Bus Creator3/1  "w"
  [w] -> Gain/1  "w"
  Bus Selector/1 -> Gain2/1  "<vcabc>"
  Unit Delay/1 -> Demux/1
  [m_filter] -> Bus Selector/1
  "abc -> dq (Power-Invariant)1"/1(dq) -> [il_dq]
  "abc -> dq (Power-Invariant)2"/1(dq) -> [ig_dq]
  "abc -> dq (Power-Invariant)"/1(dq) -> [vc_dq]
  [ig_abc] -> "PLL (iabc -> id)"/1(iabc)
  [il_dq] -> Current Controller/2(iIdq)
  [ig_dq] -> PQ Calculation (dq-Frame)/2(idq)
  PQ Calculation (dq-Frame)/1(pq) -> [pq]
  [vc_dq] -> PQ Calculation (dq-Frame)/1(vdq)
  [theta] -> "dq -> abc (Power-Invariant)"/2(theta)
  [vc_dq] -> Current Controller/3(vdq)
  Constant/1 -> Current Controller/4(enable)
  Bus Selector/2 -> Gain3/1  "<ilabc>"
  Bus Selector/3 -> Gain4/1  "<igabc>"
  [theta] -> "abc -> dq (Power-Invariant)2"/2(theta)
  [ig_abc] -> "abc -> dq (Power-Invariant)2"/1(abc)
  [il_abc] -> "abc -> dq (Power-Invariant)1"/1(abc)
  [vc_abc] -> "abc -> dq (Power-Invariant)"/1(abc)
  [theta] -> "abc -> dq (Power-Invariant)1"/2(theta)
  [theta] -> "abc -> dq (Power-Invariant)"/2(theta)
  Demux/3 -> vc/1
  Demux/2 -> vb/1
  Demux/1 -> va/1
  LCL Filter/1(m) -> [m_filter]
  Bus Creator3/1 -> m/1
  "dq -> abc (Power-Invariant)"/1(abc) -> [vi_abc]
  Current Controller/1(vidq*) -> Manual Switch/2
  Manual Switch/1 -> [vi_dq], "dq -> abc (Power-Invariant)"/1(dq)
  "PLL (iabc -> id)"/1(w) -> [w]
  "PLL (iabc -> id)"/2(theta) -> [theta]
  [vi_dq] -> PQ Calculation (dq-Frame)1/1(vdq)
  [il_dq] -> PQ Calculation (dq-Frame)1/2(idq)
  PQ Calculation (dq-Frame)1/1(pq) -> [pqi]
  [vdc] -> Bus Creator3/12  "vdc"
  Voltage Measurement/1 -> Gain7/1, Divide1/2
  [pqi] -> Demux1/1
  Demux1/1 -> Gain5/1
  Gain5/1 -> Divide1/1
  Constant2/1 -> DC Voltage Controller/3(enable)
  [vdc] -> DC Voltage Controller/2(vdc)
  Constant3/1 -> DC Voltage Controller/1(vdc*)
  Mux/1 -> Manual Switch/1, Voltage Controller/1(vcdq*)
  Constant4/1 -> Mux/1
  Divide1/1 -> Gain6/1
  Gain6/1 -> Controlled Current Source/1
  Gain7/1 -> [vdc]
  DC Voltage Controller/1(vq*) -> Gain8/1
  Gain8/1 -> Mux/2
  connections:
  LCL Filter/LConn3 -- vc/RConn1
  va/LConn1 -- vb/LConn1 -- vc/LConn1 -- LCL Filter/LConn4 -- N/RConn1
  LCL Filter/RConn3 -- c/RConn1
  LCL Filter/RConn2 -- b/RConn1
  LCL Filter/RConn1 -- a/RConn1
  LCL Filter/LConn1 -- va/RConn1
  LCL Filter/LConn2 -- vb/RConn1
  Series RLC Branch/LConn1 -- Voltage Measurement/LConn1 -- Controlled Current Source/RConn1
  Series RLC Branch/RConn1 -- Voltage Measurement/LConn2 -- Controlled Current Source/LConn1

== system SingleInverterInfBus/AC Infinite Bus (Current Type)1/PQ Calculation (dq-Frame) ==
  note: Power calculation.
      |
      | Author(s): Yitong Li
      |
      | Notes:
      |
      | The calculation is done in dq frame.
  vdq : Inport
  idq : Inport  Port=2
  Mux : Mux  Inputs=2
  Mux1 : Mux  Inputs=2
  P = vd*id+vq*iq : Fcn  Expr=u[1]*u[3]+u[2]*u[4]
  Q = -vd*iq+vq*id : Fcn  Expr=-u[1]*u[4]+u[2]*u[3]
  pq : Outport
  wires:
  Mux/1 -> pq/1
  P = vd*id+vq*iq/1 -> Mux/1
  vdq/1 -> Mux1/1
  idq/1 -> Mux1/2
  Mux1/1 -> P = vd*id+vq*iq/1, Q = -vd*iq+vq*id/1
  Q = -vd*iq+vq*id/1 -> Mux/2

== system SingleInverterInfBus/AC Infinite Bus (Current Type)1/abc -> dq (Power-Invariant) ==
  note: Frame transformation from abc to dq.
      |
      | Author(s): Yitong Li
      |
      | Notes:
      |
      | The transformation is power-invariant.
      |
      | theta is the angle that d axis leads a axis.
      |
      | q axis leads d axis by 90 degrees.
  abc : Inport
  theta : Inport  Port=2
  ->d : Fcn  Expr=cos(u(4))*u(1) + cos(u(4)-2/3*pi)*u(2) + cos(u(4)-4/3*pi)*u(3)
  ->q : Fcn  Expr=-sin(u(4))*u(1) - sin(u(4)-2/3*pi)*u(2) - sin(u(4)-4/3*pi)*u(3)
  Gain : Gain  Gain=sqrt(2/3)
  Mux5 : Mux  Inputs=2
  Mux6 : Mux  Inputs=2
  dq : Outport
  wires:
  abc/1 -> Gain/1
  ->d/1 -> Mux6/1
  Gain/1 -> Mux5/1
  theta/1 -> Mux5/2
  ->q/1 -> Mux6/2
  Mux6/1 -> dq/1
  Mux5/1 -> ->d/1, ->q/1

== system SingleInverterInfBus/AC Infinite Bus (Current Type)1/dq -> abc (Power-Invariant) ==
  note: Frame transformation from dq to abc.
      |
      | Author(s): Yitong Li
      |
      | Notes:
      |
      | The transformation is power-invariant.
      |
      | theta is the angle that dq axis leads alpha/beta axis, specifically, d axis leads alpha axis.
  dq : Inport
  theta : Inport  Port=2
  ->a : Fcn  Expr=cos(u(3))*u(1) - sin(u(3))*u(2)
  ->b : Fcn  Expr=cos(u(3)-2/3*pi)*u(1) - sin(u(3)-2/3*pi)*u(2)
  ->c : Fcn  Expr=cos(u(3)-4/3*pi)*u(1) - sin(u(3)-4/3*pi)*u(2)
  Gain : Gain  Gain=sqrt(2/3)
  Mux5 : Mux  Inputs=2
  Mux6 : Mux  Inputs=3
  abc : Outport
  wires:
  ->b/1 -> Mux6/2
  ->a/1 -> Mux6/1
  Gain/1 -> Mux5/1
  dq/1 -> Gain/1
  ->c/1 -> Mux6/3
  Mux6/1 -> abc/1
  Mux5/1 -> ->b/1, ->a/1, ->c/1
  theta/1 -> Mux5/2

== system SingleInverterInfBus/AC Infinite Bus (Current Type)2/PQ Calculation (dq-Frame) ==
  note: Power calculation.
      |
      | Author(s): Yitong Li
      |
      | Notes:
      |
      | The calculation is done in dq frame.
  vdq : Inport
  idq : Inport  Port=2
  Mux : Mux  Inputs=2
  Mux1 : Mux  Inputs=2
  P = vd*id+vq*iq : Fcn  Expr=u[1]*u[3]+u[2]*u[4]
  Q = -vd*iq+vq*id : Fcn  Expr=-u[1]*u[4]+u[2]*u[3]
  pq : Outport
  wires:
  Mux/1 -> pq/1
  P = vd*id+vq*iq/1 -> Mux/1
  vdq/1 -> Mux1/1
  idq/1 -> Mux1/2
  Mux1/1 -> P = vd*id+vq*iq/1, Q = -vd*iq+vq*id/1
  Q = -vd*iq+vq*id/1 -> Mux/2

== system SingleInverterInfBus/AC Infinite Bus (Current Type)2/abc -> dq (Power-Invariant) ==
  note: Frame transformation from abc to dq.
      |
      | Author(s): Yitong Li
      |
      | Notes:
      |
      | The transformation is power-invariant.
      |
      | theta is the angle that d axis leads a axis.
      |
      | q axis leads d axis by 90 degrees.
  abc : Inport
  theta : Inport  Port=2
  ->d : Fcn  Expr=cos(u(4))*u(1) + cos(u(4)-2/3*pi)*u(2) + cos(u(4)-4/3*pi)*u(3)
  ->q : Fcn  Expr=-sin(u(4))*u(1) - sin(u(4)-2/3*pi)*u(2) - sin(u(4)-4/3*pi)*u(3)
  Gain : Gain  Gain=sqrt(2/3)
  Mux5 : Mux  Inputs=2
  Mux6 : Mux  Inputs=2
  dq : Outport
  wires:
  abc/1 -> Gain/1
  ->d/1 -> Mux6/1
  Gain/1 -> Mux5/1
  theta/1 -> Mux5/2
  ->q/1 -> Mux6/2
  Mux6/1 -> dq/1
  Mux5/1 -> ->d/1, ->q/1

== system SingleInverterInfBus/AC Infinite Bus (Current Type)2/dq -> abc (Power-Invariant) ==
  note: Frame transformation from dq to abc.
      |
      | Author(s): Yitong Li
      |
      | Notes:
      |
      | The transformation is power-invariant.
      |
      | theta is the angle that dq axis leads alpha/beta axis, specifically, d axis leads alpha axis.
  dq : Inport
  theta : Inport  Port=2
  ->a : Fcn  Expr=cos(u(3))*u(1) - sin(u(3))*u(2)
  ->b : Fcn  Expr=cos(u(3)-2/3*pi)*u(1) - sin(u(3)-2/3*pi)*u(2)
  ->c : Fcn  Expr=cos(u(3)-4/3*pi)*u(1) - sin(u(3)-4/3*pi)*u(2)
  Gain : Gain  Gain=sqrt(2/3)
  Mux5 : Mux  Inputs=2
  Mux6 : Mux  Inputs=3
  abc : Outport
  wires:
  ->b/1 -> Mux6/2
  ->a/1 -> Mux6/1
  Gain/1 -> Mux5/1
  dq/1 -> Gain/1
  ->c/1 -> Mux6/3
  Mux6/1 -> abc/1
  Mux5/1 -> ->b/1, ->a/1, ->c/1
  theta/1 -> Mux5/2

== system SingleInverterInfBus/AC Infinite Bus (Voltage Type)1/PQ Calculation (dq-Frame)1 ==
  note: Power calculation.
      |
      | Author(s): Yitong Li
      |
      | Notes:
      |
      | The calculation is done in dq frame.
  vdq : Inport
  idq : Inport  Port=2
  Mux : Mux  Inputs=2
  Mux1 : Mux  Inputs=2
  P = vd*id+vq*iq : Fcn  Expr=u[1]*u[3]+u[2]*u[4]
  Q = -vd*iq+vq*id : Fcn  Expr=-u[1]*u[4]+u[2]*u[3]
  pq : Outport
  wires:
  Mux/1 -> pq/1
  P = vd*id+vq*iq/1 -> Mux/1
  vdq/1 -> Mux1/1
  idq/1 -> Mux1/2
  Mux1/1 -> P = vd*id+vq*iq/1, Q = -vd*iq+vq*id/1
  Q = -vd*iq+vq*id/1 -> Mux/2

== system SingleInverterInfBus/AC Infinite Bus (Voltage Type)1/abc -> dq (Power-Invariant)1 ==
  note: Frame transformation from abc to dq.
      |
      | Author(s): Yitong Li
      |
      | Notes:
      |
      | The transformation is power-invariant.
      |
      | theta is the angle that d axis leads a axis.
      |
      | q axis leads d axis by 90 degrees.
  abc : Inport
  theta : Inport  Port=2
  ->d : Fcn  Expr=cos(u(4))*u(1) + cos(u(4)-2/3*pi)*u(2) + cos(u(4)-4/3*pi)*u(3)
  ->q : Fcn  Expr=-sin(u(4))*u(1) - sin(u(4)-2/3*pi)*u(2) - sin(u(4)-4/3*pi)*u(3)
  Gain : Gain  Gain=sqrt(2/3)
  Mux5 : Mux  Inputs=2
  Mux6 : Mux  Inputs=2
  dq : Outport
  wires:
  abc/1 -> Gain/1
  ->d/1 -> Mux6/1
  Gain/1 -> Mux5/1
  theta/1 -> Mux5/2
  ->q/1 -> Mux6/2
  Mux6/1 -> dq/1
  Mux5/1 -> ->d/1, ->q/1

== system SingleInverterInfBus/AC Infinite Bus (Voltage Type)1/dq -> abc (Power-Invariant)1 ==
  note: Frame transformation from dq to abc.
      |
      | Author(s): Yitong Li
      |
      | Notes:
      |
      | The transformation is power-invariant.
      |
      | theta is the angle that dq axis leads alpha/beta axis, specifically, d axis leads alpha axis.
  dq : Inport
  theta : Inport  Port=2
  ->a : Fcn  Expr=cos(u(3))*u(1) - sin(u(3))*u(2)
  ->b : Fcn  Expr=cos(u(3)-2/3*pi)*u(1) - sin(u(3)-2/3*pi)*u(2)
  ->c : Fcn  Expr=cos(u(3)-4/3*pi)*u(1) - sin(u(3)-4/3*pi)*u(2)
  Gain : Gain  Gain=sqrt(2/3)
  Mux5 : Mux  Inputs=2
  Mux6 : Mux  Inputs=3
  abc : Outport
  wires:
  ->b/1 -> Mux6/2
  ->a/1 -> Mux6/1
  Gain/1 -> Mux5/1
  dq/1 -> Gain/1
  ->c/1 -> Mux6/3
  Mux6/1 -> abc/1
  Mux5/1 -> ->b/1, ->a/1, ->c/1
  theta/1 -> Mux5/2

== system SingleInverterInfBus/AC Infinite Bus (Voltage Type)2/PQ Calculation (dq-Frame)1 ==
  note: Power calculation.
      |
      | Author(s): Yitong Li
      |
      | Notes:
      |
      | The calculation is done in dq frame.
  vdq : Inport
  idq : Inport  Port=2
  Mux : Mux  Inputs=2
  Mux1 : Mux  Inputs=2
  P = vd*id+vq*iq : Fcn  Expr=u[1]*u[3]+u[2]*u[4]
  Q = -vd*iq+vq*id : Fcn  Expr=-u[1]*u[4]+u[2]*u[3]
  pq : Outport
  wires:
  Mux/1 -> pq/1
  P = vd*id+vq*iq/1 -> Mux/1
  vdq/1 -> Mux1/1
  idq/1 -> Mux1/2
  Mux1/1 -> P = vd*id+vq*iq/1, Q = -vd*iq+vq*id/1
  Q = -vd*iq+vq*id/1 -> Mux/2

== system SingleInverterInfBus/AC Infinite Bus (Voltage Type)2/abc -> dq (Power-Invariant)1 ==
  note: Frame transformation from abc to dq.
      |
      | Author(s): Yitong Li
      |
      | Notes:
      |
      | The transformation is power-invariant.
      |
      | theta is the angle that d axis leads a axis.
      |
      | q axis leads d axis by 90 degrees.
  abc : Inport
  theta : Inport  Port=2
  ->d : Fcn  Expr=cos(u(4))*u(1) + cos(u(4)-2/3*pi)*u(2) + cos(u(4)-4/3*pi)*u(3)
  ->q : Fcn  Expr=-sin(u(4))*u(1) - sin(u(4)-2/3*pi)*u(2) - sin(u(4)-4/3*pi)*u(3)
  Gain : Gain  Gain=sqrt(2/3)
  Mux5 : Mux  Inputs=2
  Mux6 : Mux  Inputs=2
  dq : Outport
  wires:
  abc/1 -> Gain/1
  ->d/1 -> Mux6/1
  Gain/1 -> Mux5/1
  theta/1 -> Mux5/2
  ->q/1 -> Mux6/2
  Mux6/1 -> dq/1
  Mux5/1 -> ->d/1, ->q/1

== system SingleInverterInfBus/AC Infinite Bus (Voltage Type)2/dq -> abc (Power-Invariant)1 ==
  note: Frame transformation from dq to abc.
      |
      | Author(s): Yitong Li
      |
      | Notes:
      |
      | The transformation is power-invariant.
      |
      | theta is the angle that dq axis leads alpha/beta axis, specifically, d axis leads alpha axis.
  dq : Inport
  theta : Inport  Port=2
  ->a : Fcn  Expr=cos(u(3))*u(1) - sin(u(3))*u(2)
  ->b : Fcn  Expr=cos(u(3)-2/3*pi)*u(1) - sin(u(3)-2/3*pi)*u(2)
  ->c : Fcn  Expr=cos(u(3)-4/3*pi)*u(1) - sin(u(3)-4/3*pi)*u(2)
  Gain : Gain  Gain=sqrt(2/3)
  Mux5 : Mux  Inputs=2
  Mux6 : Mux  Inputs=3
  abc : Outport
  wires:
  ->b/1 -> Mux6/2
  ->a/1 -> Mux6/1
  Gain/1 -> Mux5/1
  dq/1 -> Gain/1
  ->c/1 -> Mux6/3
  Mux6/1 -> abc/1
  Mux5/1 -> ->b/1, ->a/1, ->c/1
  theta/1 -> Mux5/2

== system SingleInverterInfBus/AC Infinite Bus (Voltage Type)3/PQ Calculation (dq-Frame)1 ==
  note: Power calculation.
      |
      | Author(s): Yitong Li
      |
      | Notes:
      |
      | The calculation is done in dq frame.
  vdq : Inport
  idq : Inport  Port=2
  Mux : Mux  Inputs=2
  Mux1 : Mux  Inputs=2
  P = vd*id+vq*iq : Fcn  Expr=u[1]*u[3]+u[2]*u[4]
  Q = -vd*iq+vq*id : Fcn  Expr=-u[1]*u[4]+u[2]*u[3]
  pq : Outport
  wires:
  Mux/1 -> pq/1
  P = vd*id+vq*iq/1 -> Mux/1
  vdq/1 -> Mux1/1
  idq/1 -> Mux1/2
  Mux1/1 -> P = vd*id+vq*iq/1, Q = -vd*iq+vq*id/1
  Q = -vd*iq+vq*id/1 -> Mux/2

== system SingleInverterInfBus/AC Infinite Bus (Voltage Type)3/abc -> dq (Power-Invariant)1 ==
  note: Frame transformation from abc to dq.
      |
      | Author(s): Yitong Li
      |
      | Notes:
      |
      | The transformation is power-invariant.
      |
      | theta is the angle that d axis leads a axis.
      |
      | q axis leads d axis by 90 degrees.
  abc : Inport
  theta : Inport  Port=2
  ->d : Fcn  Expr=cos(u(4))*u(1) + cos(u(4)-2/3*pi)*u(2) + cos(u(4)-4/3*pi)*u(3)
  ->q : Fcn  Expr=-sin(u(4))*u(1) - sin(u(4)-2/3*pi)*u(2) - sin(u(4)-4/3*pi)*u(3)
  Gain : Gain  Gain=sqrt(2/3)
  Mux5 : Mux  Inputs=2
  Mux6 : Mux  Inputs=2
  dq : Outport
  wires:
  abc/1 -> Gain/1
  ->d/1 -> Mux6/1
  Gain/1 -> Mux5/1
  theta/1 -> Mux5/2
  ->q/1 -> Mux6/2
  Mux6/1 -> dq/1
  Mux5/1 -> ->d/1, ->q/1

== system SingleInverterInfBus/AC Infinite Bus (Voltage Type)3/dq -> abc (Power-Invariant)1 ==
  note: Frame transformation from dq to abc.
      |
      | Author(s): Yitong Li
      |
      | Notes:
      |
      | The transformation is power-invariant.
      |
      | theta is the angle that dq axis leads alpha/beta axis, specifically, d axis leads alpha axis.
  dq : Inport
  theta : Inport  Port=2
  ->a : Fcn  Expr=cos(u(3))*u(1) - sin(u(3))*u(2)
  ->b : Fcn  Expr=cos(u(3)-2/3*pi)*u(1) - sin(u(3)-2/3*pi)*u(2)
  ->c : Fcn  Expr=cos(u(3)-4/3*pi)*u(1) - sin(u(3)-4/3*pi)*u(2)
  Gain : Gain  Gain=sqrt(2/3)
  Mux5 : Mux  Inputs=2
  Mux6 : Mux  Inputs=3
  abc : Outport
  wires:
  ->b/1 -> Mux6/2
  ->a/1 -> Mux6/1
  Gain/1 -> Mux5/1
  dq/1 -> Gain/1
  ->c/1 -> Mux6/3
  Mux6/1 -> abc/1
  Mux5/1 -> ->b/1, ->a/1, ->c/1
  theta/1 -> Mux5/2

== system SingleInverterInfBus/AC Infinite Bus (Voltage Type)4/PQ Calculation (dq-Frame)1 ==
  note: Power calculation.
      |
      | Author(s): Yitong Li
      |
      | Notes:
      |
      | The calculation is done in dq frame.
  vdq : Inport
  idq : Inport  Port=2
  Mux : Mux  Inputs=2
  Mux1 : Mux  Inputs=2
  P = vd*id+vq*iq : Fcn  Expr=u[1]*u[3]+u[2]*u[4]
  Q = -vd*iq+vq*id : Fcn  Expr=-u[1]*u[4]+u[2]*u[3]
  pq : Outport
  wires:
  Mux/1 -> pq/1
  P = vd*id+vq*iq/1 -> Mux/1
  vdq/1 -> Mux1/1
  idq/1 -> Mux1/2
  Mux1/1 -> P = vd*id+vq*iq/1, Q = -vd*iq+vq*id/1
  Q = -vd*iq+vq*id/1 -> Mux/2

== system SingleInverterInfBus/AC Infinite Bus (Voltage Type)4/abc -> dq (Power-Invariant)1 ==
  note: Frame transformation from abc to dq.
      |
      | Author(s): Yitong Li
      |
      | Notes:
      |
      | The transformation is power-invariant.
      |
      | theta is the angle that d axis leads a axis.
      |
      | q axis leads d axis by 90 degrees.
  abc : Inport
  theta : Inport  Port=2
  ->d : Fcn  Expr=cos(u(4))*u(1) + cos(u(4)-2/3*pi)*u(2) + cos(u(4)-4/3*pi)*u(3)
  ->q : Fcn  Expr=-sin(u(4))*u(1) - sin(u(4)-2/3*pi)*u(2) - sin(u(4)-4/3*pi)*u(3)
  Gain : Gain  Gain=sqrt(2/3)
  Mux5 : Mux  Inputs=2
  Mux6 : Mux  Inputs=2
  dq : Outport
  wires:
  abc/1 -> Gain/1
  ->d/1 -> Mux6/1
  Gain/1 -> Mux5/1
  theta/1 -> Mux5/2
  ->q/1 -> Mux6/2
  Mux6/1 -> dq/1
  Mux5/1 -> ->d/1, ->q/1

== system SingleInverterInfBus/AC Infinite Bus (Voltage Type)4/dq -> abc (Power-Invariant)1 ==
  note: Frame transformation from dq to abc.
      |
      | Author(s): Yitong Li
      |
      | Notes:
      |
      | The transformation is power-invariant.
      |
      | theta is the angle that dq axis leads alpha/beta axis, specifically, d axis leads alpha axis.
  dq : Inport
  theta : Inport  Port=2
  ->a : Fcn  Expr=cos(u(3))*u(1) - sin(u(3))*u(2)
  ->b : Fcn  Expr=cos(u(3)-2/3*pi)*u(1) - sin(u(3)-2/3*pi)*u(2)
  ->c : Fcn  Expr=cos(u(3)-4/3*pi)*u(1) - sin(u(3)-4/3*pi)*u(2)
  Gain : Gain  Gain=sqrt(2/3)
  Mux5 : Mux  Inputs=2
  Mux6 : Mux  Inputs=3
  abc : Outport
  wires:
  ->b/1 -> Mux6/2
  ->a/1 -> Mux6/1
  Gain/1 -> Mux5/1
  dq/1 -> Gain/1
  ->c/1 -> Mux6/3
  Mux6/1 -> abc/1
  Mux5/1 -> ->b/1, ->a/1, ->c/1
  theta/1 -> Mux5/2

== system SingleInverterInfBus/AC Infinite Bus (Voltage Type)5/PQ Calculation (dq-Frame)1 ==
  note: Power calculation.
      |
      | Author(s): Yitong Li
      |
      | Notes:
      |
      | The calculation is done in dq frame.
  vdq : Inport
  idq : Inport  Port=2
  Mux : Mux  Inputs=2
  Mux1 : Mux  Inputs=2
  P = vd*id+vq*iq : Fcn  Expr=u[1]*u[3]+u[2]*u[4]
  Q = -vd*iq+vq*id : Fcn  Expr=-u[1]*u[4]+u[2]*u[3]
  pq : Outport
  wires:
  Mux/1 -> pq/1
  P = vd*id+vq*iq/1 -> Mux/1
  vdq/1 -> Mux1/1
  idq/1 -> Mux1/2
  Mux1/1 -> P = vd*id+vq*iq/1, Q = -vd*iq+vq*id/1
  Q = -vd*iq+vq*id/1 -> Mux/2

== system SingleInverterInfBus/AC Infinite Bus (Voltage Type)5/abc -> dq (Power-Invariant)1 ==
  note: Frame transformation from abc to dq.
      |
      | Author(s): Yitong Li
      |
      | Notes:
      |
      | The transformation is power-invariant.
      |
      | theta is the angle that d axis leads a axis.
      |
      | q axis leads d axis by 90 degrees.
  abc : Inport
  theta : Inport  Port=2
  ->d : Fcn  Expr=cos(u(4))*u(1) + cos(u(4)-2/3*pi)*u(2) + cos(u(4)-4/3*pi)*u(3)
  ->q : Fcn  Expr=-sin(u(4))*u(1) - sin(u(4)-2/3*pi)*u(2) - sin(u(4)-4/3*pi)*u(3)
  Gain : Gain  Gain=sqrt(2/3)
  Mux5 : Mux  Inputs=2
  Mux6 : Mux  Inputs=2
  dq : Outport
  wires:
  abc/1 -> Gain/1
  ->d/1 -> Mux6/1
  Gain/1 -> Mux5/1
  theta/1 -> Mux5/2
  ->q/1 -> Mux6/2
  Mux6/1 -> dq/1
  Mux5/1 -> ->d/1, ->q/1

== system SingleInverterInfBus/AC Infinite Bus (Voltage Type)5/dq -> abc (Power-Invariant)1 ==
  note: Frame transformation from dq to abc.
      |
      | Author(s): Yitong Li
      |
      | Notes:
      |
      | The transformation is power-invariant.
      |
      | theta is the angle that dq axis leads alpha/beta axis, specifically, d axis leads alpha axis.
  dq : Inport
  theta : Inport  Port=2
  ->a : Fcn  Expr=cos(u(3))*u(1) - sin(u(3))*u(2)
  ->b : Fcn  Expr=cos(u(3)-2/3*pi)*u(1) - sin(u(3)-2/3*pi)*u(2)
  ->c : Fcn  Expr=cos(u(3)-4/3*pi)*u(1) - sin(u(3)-4/3*pi)*u(2)
  Gain : Gain  Gain=sqrt(2/3)
  Mux5 : Mux  Inputs=2
  Mux6 : Mux  Inputs=3
  abc : Outport
  wires:
  ->b/1 -> Mux6/2
  ->a/1 -> Mux6/1
  Gain/1 -> Mux5/1
  dq/1 -> Gain/1
  ->c/1 -> Mux6/3
  Mux6/1 -> abc/1
  Mux5/1 -> ->b/1, ->a/1, ->c/1
  theta/1 -> Mux5/2

== system SingleInverterInfBus/AC Infinite Bus (Voltage Type)6/PQ Calculation (dq-Frame)1 ==
  note: Power calculation.
      |
      | Author(s): Yitong Li
      |
      | Notes:
      |
      | The calculation is done in dq frame.
  vdq : Inport
  idq : Inport  Port=2
  Mux : Mux  Inputs=2
  Mux1 : Mux  Inputs=2
  P = vd*id+vq*iq : Fcn  Expr=u[1]*u[3]+u[2]*u[4]
  Q = -vd*iq+vq*id : Fcn  Expr=-u[1]*u[4]+u[2]*u[3]
  pq : Outport
  wires:
  Mux/1 -> pq/1
  P = vd*id+vq*iq/1 -> Mux/1
  vdq/1 -> Mux1/1
  idq/1 -> Mux1/2
  Mux1/1 -> P = vd*id+vq*iq/1, Q = -vd*iq+vq*id/1
  Q = -vd*iq+vq*id/1 -> Mux/2

== system SingleInverterInfBus/AC Infinite Bus (Voltage Type)6/abc -> dq (Power-Invariant)1 ==
  note: Frame transformation from abc to dq.
      |
      | Author(s): Yitong Li
      |
      | Notes:
      |
      | The transformation is power-invariant.
      |
      | theta is the angle that d axis leads a axis.
      |
      | q axis leads d axis by 90 degrees.
  abc : Inport
  theta : Inport  Port=2
  ->d : Fcn  Expr=cos(u(4))*u(1) + cos(u(4)-2/3*pi)*u(2) + cos(u(4)-4/3*pi)*u(3)
  ->q : Fcn  Expr=-sin(u(4))*u(1) - sin(u(4)-2/3*pi)*u(2) - sin(u(4)-4/3*pi)*u(3)
  Gain : Gain  Gain=sqrt(2/3)
  Mux5 : Mux  Inputs=2
  Mux6 : Mux  Inputs=2
  dq : Outport
  wires:
  abc/1 -> Gain/1
  ->d/1 -> Mux6/1
  Gain/1 -> Mux5/1
  theta/1 -> Mux5/2
  ->q/1 -> Mux6/2
  Mux6/1 -> dq/1
  Mux5/1 -> ->d/1, ->q/1
